simulink model "part4_implement_starter"  (R2024b)
settings: Solver=ode1  StartTime=0.0  StopTime=400  FixedStep=.002  RelTol=1e-3  EnableMultiTasking=on
InitFcn:
  | StartStop___PWM = 1
libraries: c2837xDlib x2, fricblocks x1, ece486lib x1
settings Model: SimulationMode=external  ExtModeTrigDuration=8  Creator=The MathWorks, Inc.  LastModifiedBy=fve2
settings SolverCC: AlgebraicLoopSolver=TrustRegion  MaxZcPerStep=1
settings OptimizationCC: DefaultUnderspecifiedDataType=single  EnhancedBackFolding=on  PassReuseOutputArgsAs=Individual arguments  MaxStackSize=1024  OptimizeBlockOrder=speed  DifferentSizesBufferReuse=on  OptimizationCustomize=off  EfficientTunableParamExpr=on
settings DebuggingCC: ParameterTunabilityLossMsg=error  UnconnectedInputMsg=warning  UnconnectedOutputMsg=warning  UnconnectedLineMsg=warning
settings HardwareCC: ProdBitPerChar=16  ProdBitPerInt=16  ProdBitPerPointer=32  ProdBitPerSizeT=32  ProdBitPerPtrDiffT=32  ProdLargestAtomicInteger=Integer  ProdLargestAtomicFloat=None  ProdWordSize=16  ProdLongLongMode=on  ProdHWDeviceType=Texas Instruments->C2000
settings ModelReferenceCC: EnableRefExpFcnMdlSchedulingChecks=on
settings SFSimCC: MATLABDynamicMemAlloc=off
settings RTWCC: Description=Embedded Coder  SystemTargetFile=ert.tlc  HardwareBoard=TI Delfino F28379D LaunchPad  TemplateMakefile=ert_default_tmf  GenerateReport=on  Toolchain=Texas Instruments Code Composer Studio (C2000)  GPUComputeCapability=3.5  DLArmComputeVersion=19.05
settings CodeAppCC: ForceParamTrailComments=on  IgnoreCustomStorageClasses=off  OperatorAnnotations=on  SimulinkDataObjDesc=on  SFDataObjDesc=on  InsertBlockDesc=on
settings ERTTargetCC: CodeReplacementLibrary=TI C28x  SupportContinuousTime=on  ExtModeStaticAllocSize=10000  InlinedParameterPlacement=Hierarchical  DynamicArrayContainerType=coder::array

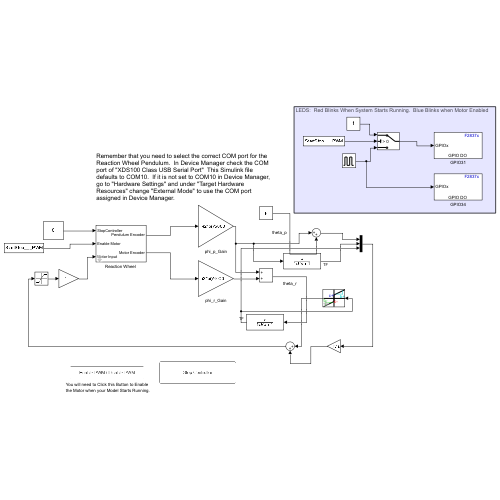
[thumbnail: Simulink's stored preview of the top-level diagram]
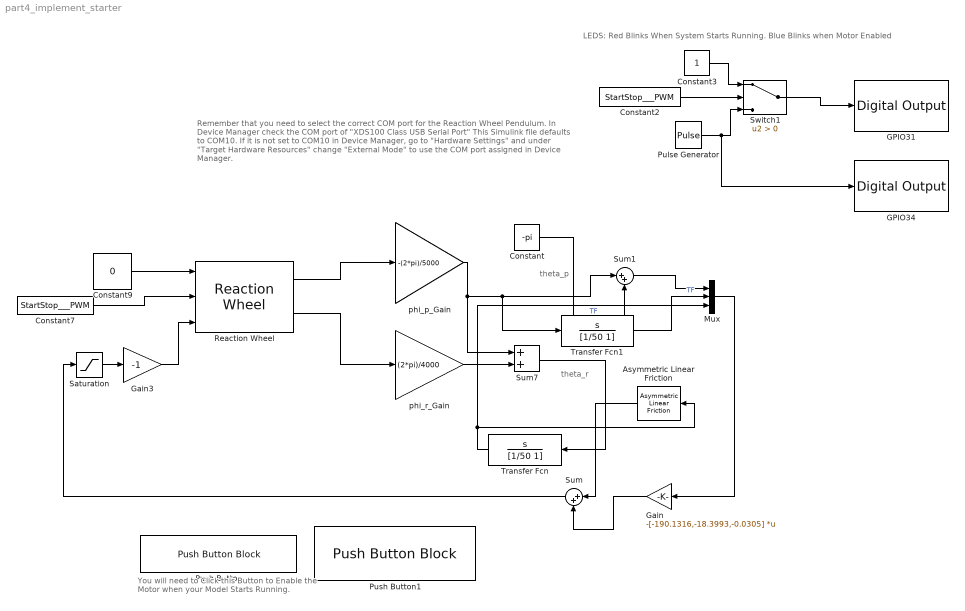
== system part4_implement_starter ==
  note: theta_r
  note: theta_p
  note: Remember that you need to select the correct COM port for the Reaction Wheel Pendulum. In Device Manager check the COM port of "XDS100 Class USB Serial Port" This Simulink file defaults to COM10. If it is not set to COM10 in Device Manager, go to "Hardware Settings" and under "Target Hardware Resources" change "External Mode" to use the COM port assigned in Device Manager.
  note: You will need to Click this Button to Enable
      | the Motor when your Model Starts Running.
  note: LEDS: Red Blinks When System Starts Running. Blue Blinks when Motor Enabled
  Asymmetric Linear Friction : fricblocks/Asymmetric  Linear Friction  intercept1=.05  intercept2=-.05  slope1=0.08  slope2=0.08
  Constant : Constant  Value=-pi
  Constant2 : Constant  Value=StartStop___PWM
  Constant3 : Constant
  Constant7 : Constant  Value=StartStop___PWM
  Constant9 : Constant  Value=0
  GPIO31 : c2837xDlib/Digital Output  GPIO_Number=GPIO24~GPIO31  GPIO_Bit0=off  GPIO_BIT0_Toggle=off  GPIO_Bit1=off  GPIO_BIT1_Toggle=off  GPIO_Bit2=off  GPIO_BIT2_Toggle=off  GPIO_Bit3=off  GPIO_BIT3_Toggle=off  GPIO_Bit4=off  GPIO_BIT4_Toggle=off  GPIO_Bit5=off  GPIO_BIT5_Toggle=off  GPIO_Bit6=off  GPIO_BIT6_Toggle=off  GPIO_Bit7=on  GPIO_BIT7_Toggle=off
  GPIO34 : c2837xDlib/Digital Output  GPIO_Number=GPIO32~GPIO39  GPIO_Bit0=off  GPIO_BIT0_Toggle=off  GPIO_Bit1=off  GPIO_BIT1_Toggle=off  GPIO_Bit2=on  GPIO_BIT2_Toggle=off  GPIO_Bit3=off  GPIO_BIT3_Toggle=off  GPIO_Bit4=off  GPIO_BIT4_Toggle=off  GPIO_Bit5=off  GPIO_BIT5_Toggle=off  GPIO_Bit6=off  GPIO_BIT6_Toggle=off  GPIO_Bit7=off  GPIO_BIT7_Toggle=off
  Gain : Gain  Gain=-[-190.1316,-18.3993,-0.0305]  Multiplication=Matrix(K*u)
  Gain3 : Gain  Gain=-1  SaturateOnIntegerOverflow=on  OutDataTypeStr=Inherit: Same as input  ParamDataTypeStr=Inherit: Same as input
  Mux : Mux  Inputs=3
  Pulse Generator : DiscretePulseGenerator  PulseType=Time based  Period=1  PulseWidth=50
  Push Button : PushButtonBlock  ButtonText=Enable PWM / Disable PWM  OnValue=0  ButtonType=Latch  OffValue=1.000000
  Push Button1 : PushButtonBlock  ButtonText=Stop Controller  OffValue=0.000000
  "Reaction Wheel " : ece486lib/Reaction Wheel  SampleTime=.002
  Saturation : Saturate  UpperLimit=10  LowerLimit=-10
  Sum : Sum  Inputs=|++
  Sum1 : Sum  Inputs=|++
  Sum7 : Sum  InputSameDT=on  SaturateOnIntegerOverflow=on  OutDataTypeStr=Inherit: Same as first input
  Switch1 : Switch  Criteria=u2 > Threshold  SaturateOnIntegerOverflow=off  InputSameDT=off
  Transfer Fcn : TransferFcn  Numerator=[1 0]  Denominator=[1/50 1]
  Transfer Fcn1 : TransferFcn  Numerator=[1 0]  Denominator=[1/50 1]
  phi_p_Gain : Gain  Gain=-(2*pi)/5000  SaturateOnIntegerOverflow=on  OutDataTypeStr=Inherit: Same as input  ParamDataTypeStr=Inherit: Same as input
  phi_r_Gain : Gain  Gain=(2*pi)/4000  SaturateOnIntegerOverflow=on  OutDataTypeStr=Inherit: Same as input  ParamDataTypeStr=Inherit: Same as input
  wires:
  phi_r_Gain/1 -> Sum7/2
  Constant9/1 -> "Reaction Wheel "/1
  Gain3/1 -> "Reaction Wheel "/3
  Constant7/1 -> "Reaction Wheel "/2
  "Reaction Wheel "/1 -> phi_p_Gain/1
  "Reaction Wheel "/2 -> phi_r_Gain/1
  Pulse Generator/1 -> GPIO34/1, Switch1/3
  Switch1/1 -> GPIO31/1
  Constant3/1 -> Switch1/1
  Constant2/1 -> Switch1/2
  Sum7/1 -> Transfer Fcn/1
  Transfer Fcn/1 -> Mux/3, Asymmetric Linear Friction/1  "TF"
  Mux/1 -> Gain/1
  Constant/1 -> Sum1/2
  phi_p_Gain/1 -> Transfer Fcn1/1, Sum1/1, Sum7/1
  Sum1/1 -> Mux/1
  Transfer Fcn1/1 -> Mux/2  "TF"
  Saturation/1 -> Gain3/1
  Gain/1 -> Sum/2
  Asymmetric Linear Friction/1 -> Sum/1
  Sum/1 -> Saturation/1
